simulink model "ControlDC_Velocidad_RTWT"  (Simulink 7.6)
settings: Solver=ode5  StartTime=0.0  StopTime=inf  FixedStep=T  RelTol=1e-3
undefined symbols (not defined in the file or in its folder): National_Instruments, PCI, T
libraries: rtwinlib x3, simulink x1, simulink_need_slupdate x1
settings Model: Creator=Rafa  LastModifiedBy=Rafa  SimulationMode=external
settings HardwareCC: ProdIntDivRoundTo=Zero  ProdEndianess=LittleEndian  ProdHWDeviceType=Generic->32-bit x86 compatible
settings RTWCC: SystemTargetFile=rtwin.tlc  TemplateMakefile=rtwin.tmf  Description=Real-Time Windows Target  ProcessScript=rtwin_make_rtw_hook  RTWCompilerOptimization=On
settings CodeAppCC: MaxIdLength=95
settings RTWinTargetCC: TargetLibSuffix=_rtwin.lib  TargetPreCompLibLocation=G:\ProgramasXP\MatlabR2010b\toolbox\rtw\targets\rtwin\lib\win32  TargetFunctionLibrary=ANSI_C  ERTCodeCoverageTool=None  PortableWordSizes=off

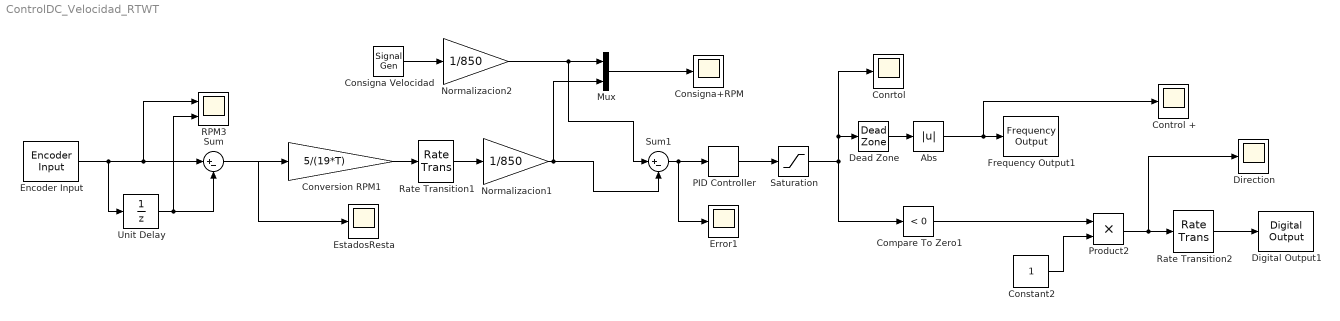
== system ControlDC_Velocidad_RTWT ==
  Abs : Abs
  Compare To Zero1 : simulink/Logic and Bit Operations/Compare To Zero  SystemSampleTime=-1  relop=<  LogicOutDataTypeMode=uint8
  Conrtol : Scope
      settings: TimeRange=100  YMin=-1.5  YMax=1.5  DataFormat=Structure
  Consigna Velocidad : SignalGenerator  WaveForm=square  Amplitude=800  Frequency=0.3
  Consigna+RPM : Scope
      settings: YMin=-1  YMax=1  SaveName=ScopeData2
  Constant2 : Constant
  Control + : Scope
      settings: TimeRange=100  YMin=-1.5  YMax=1.5  SaveName=ScopeData3  DataFormat=Structure
  Conversion RPM1 : Gain  Gain=5/(19*T)
  Dead Zone : DeadZone  LowerValue=-0.1  UpperValue=0.1  SaturateOnIntegerOverflow=on
  Digital Output1 : rtwinlib/Digital Output  SampleTime=T  DrvName=National_Instruments/PCI-6221  DrvAddress=4294967295  DrvOptions=[1 1 20480 3 1]  Channels=1  BitMode=1  InitialValue=0  FinalValue=0
      settings: AttributesFormatString=National Instruments\nPCI-6221 [auto]
  Direction : Scope
      settings: TimeRange=100  YMin=-1.5  YMax=1.5  DataFormat=Structure
  Encoder Input : rtwinlib/Encoder Input  SampleTime=T  DrvName=National_Instruments/PCI-6221  DrvAddress=4294967295  DrvOptions=[1 1 20480 3 2]  Channels=2  QuadMode=3  IndexPulse=1  InputFilter=Inf  DataType=1
      settings: AttributesFormatString=National Instruments\nPCI-6221 [auto]
  Error1 : Scope
      settings: SaveName=ScopeData7
  EstadosResta : Scope
      settings: TimeRange=100  YMin=-35  YMax=35  SaveName=ScopeData4  DataFormat=Structure  MaxDataPoints=100000
  Frequency Output1 : rtwinlib/Frequency Output  SampleTime=-1  DrvName=National_Instruments/PCI-6221  DrvAddress=4294967295  DrvOptions=[1 1 20480 3 1]  Channels=1  FrequencySource=1  Frequency=1/T  FrequencyFinalValue=[]  DutySource=2  Duty=0  DutyFinalValue=0
      settings: AttributesFormatString=National Instruments\nPCI-6221 [auto]
  Mux : Mux  Inputs=2
  Normalizacion1 : Gain  Gain=1/850
  Normalizacion2 : Gain  Gain=1/850
  PID Controller : simulink_need_slupdate/PID Controller  SystemSampleTime=-1  P=4  I=40  D=0.08
  Product2 : Product  RndMeth=Zero
  RPM3 : Scope  NumInputPorts=2
      settings: TimeRange=100  YMin=0~0  YMax=3500~3500  SaveName=ScopeData6  DataFormat=Structure  MaxDataPoints=100000
  Rate Transition1 : RateTransition  OutPortSampleTime=T
  Rate Transition2 : RateTransition  OutPortSampleTime=T
  Saturation : Saturate  UpperLimit=1  LowerLimit=-1
  Sum : Sum  Inputs=|+-
  Sum1 : Sum  Inputs=|+-
  Unit Delay : UnitDelay  SampleTime=T
  wires:
  Product2/1 -> Rate Transition2/1, Direction/1
  Compare To Zero1/1 -> Product2/1
  Constant2/1 -> Product2/2
  Abs/1 -> Frequency Output1/1, Control +/1
  Saturation/1 -> Conrtol/1, Dead Zone/1, Compare To Zero1/1
  Rate Transition2/1 -> Digital Output1/1
  Consigna Velocidad/1 -> Normalizacion2/1
  Sum1/1 -> PID Controller/1, Error1/1
  Normalizacion2/1 -> Mux/1, Sum1/1
  PID Controller/1 -> Saturation/1
  Mux/1 -> Consigna+RPM/1
  Encoder Input/1 -> RPM3/1, Sum/1, Unit Delay/1
  Unit Delay/1 -> RPM3/2, Sum/2
  Sum/1 -> EstadosResta/1, Conversion RPM1/1
  Conversion RPM1/1 -> Rate Transition1/1
  Normalizacion1/1 -> Mux/2, Sum1/2
  Dead Zone/1 -> Abs/1
  Rate Transition1/1 -> Normalizacion1/1
